simulink model "Controlador"  (Simulink 7.3)
settings: Solver=ode45  StartTime=0.0  StopTime=10  MaxStep=0.03  MinStep=0.01  RelTol=1e-3
values from neighbouring files (symbols this model uses):
  K = lqr(A,B,Q,R)    [LQR.m]
settings Model: Creator=Daniel  LastModifiedBy=Daniel
settings SolverCC: InitialStep=0.01

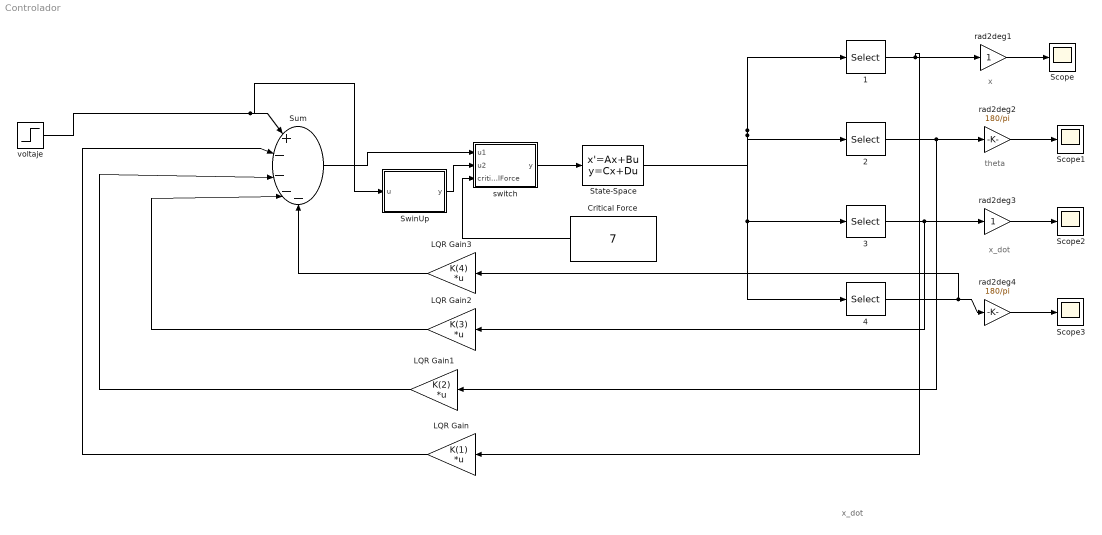
== system Controlador ==
  note: x
  note: theta
  note: x_dot
  note: x_dot
  " 1" : Selector  InputPortWidth=4  IndexOptions=Index vector (dialog)  Indices=1  OutputSizes=1
  " 2" : Selector  InputPortWidth=4  IndexOptions=Index vector (dialog)  Indices=2  OutputSizes=1
  " 3" : Selector  InputPortWidth=4  IndexOptions=Index vector (dialog)  Indices=3  OutputSizes=1
  " 4" : Selector  InputPortWidth=4  IndexOptions=Index vector (dialog)  Indices=4  OutputSizes=1
  Critical Force : Constant  Value=7  OutDataType=fixdt(1, 16)  OutScaling=2^0
  LQR Gain : Gain  Gain=K(1)  Multiplication=Matrix(K*u)  SaturateOnIntegerOverflow=on  OutDataTypeStr=Inherit: Same as input  ParamDataTypeStr=Inherit: Same as input
  LQR Gain1 : Gain  Gain=K(2)  Multiplication=Matrix(K*u)  SaturateOnIntegerOverflow=on  OutDataTypeStr=Inherit: Same as input  ParamDataTypeStr=Inherit: Same as input
  LQR Gain2 : Gain  Gain=K(3)  Multiplication=Matrix(K*u)  SaturateOnIntegerOverflow=on  OutDataTypeStr=Inherit: Same as input  ParamDataTypeStr=Inherit: Same as input
  LQR Gain3 : Gain  Gain=K(4)  Multiplication=Matrix(K*u)  SaturateOnIntegerOverflow=on  OutDataTypeStr=Inherit: Same as input  ParamDataTypeStr=Inherit: Same as input
  Scope{,1..3} (4 alike) : Scope
      Scope2 settings: SaveName=ScopeData2
      Scope3 settings: SaveName=ScopeData3
  State-Space : StateSpace  A="[0 0 1 0; 0 0 0 1; 0 0.5401 -0.7235 0; 0  14.955 -0.9854 0]"  B="[0  ;0 ;2.2747 ;3.0978]"  C=eye(4)  D=[0;0;0;0]  X0=[ 0 ; 0; 0; 0 ]
  Sum : Sum  Inputs=|+----  OutDataType=fixdt(1, 16)  OutScaling=2^0
  SwinUp : Stateflow chart
  rad2deg1 : Gain  SaturateOnIntegerOverflow=on  OutDataTypeStr=Inherit: Same as input  ParamDataTypeStr=Inherit: Same as input
  rad2deg2 : Gain  Gain=180/pi  SaturateOnIntegerOverflow=on  OutDataTypeStr=Inherit: Same as input  ParamDataTypeStr=Inherit: Same as input
  rad2deg3 : Gain  SaturateOnIntegerOverflow=on  OutDataTypeStr=Inherit: Same as input  ParamDataTypeStr=Inherit: Same as input
  rad2deg4 : Gain  Gain=180/pi  SaturateOnIntegerOverflow=on  OutDataTypeStr=Inherit: Same as input  ParamDataTypeStr=Inherit: Same as input
  switch : Stateflow chart
  voltaje : Step  Time=0  After=5  SampleTime=0
  wires:
  " 1"/1 -> rad2deg1/1, LQR Gain/1
  " 2"/1 -> rad2deg2/1, LQR Gain1/1
  " 3"/1 -> rad2deg3/1, LQR Gain2/1
  rad2deg4/1 -> Scope3/1
  rad2deg3/1 -> Scope2/1
  rad2deg2/1 -> Scope1/1
  rad2deg1/1 -> Scope/1
  LQR Gain/1 -> Sum/2
  LQR Gain1/1 -> Sum/3
  LQR Gain2/1 -> Sum/4
  LQR Gain3/1 -> Sum/5
  State-Space/1 -> " 1"/1, " 2"/1, " 3"/1, " 4"/1
  " 4"/1 -> rad2deg4/1, LQR Gain3/1
  voltaje/1 -> Sum/1, SwinUp/1(u)
  Sum/1 -> switch/1(u1)
  switch/1(y) -> State-Space/1
  SwinUp/1(y) -> switch/2(u2)
  Critical Force/1 -> switch/3(criticalForce)

== matlab function switch ==
  data: u1 input double; y output double; u2 input double; criticalForce input double
function y = fcn(u1,u2,criticalForce)
%#eml
if (abs(u2) < criticalForce)
    y = u2;
else
    y = u1;
end

== matlab function SwinUp ==
  data: u input double; y output double
function y = fcn(u)
%#eml
%y = sin(u);
y=exp(2)*sin(u);
end
